simulink model "Grav_VarAeroBlock"  (R2016b)
settings: Solver=VariableStepAuto  StartTime=0.0  StopTime=10.0  RelTol=1e-3
undefined symbols (not defined in the file or in its folder): Sim
libraries: aerolibgravity2 x1
settings Model: Creator=rega0051  LastModifiedBy=rega0051
settings DataIOCC: SaveOutput=off  SignalLogging=off  DSMLogging=off  SaveTime=off

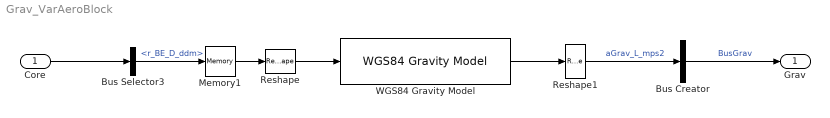
== system Grav_VarAeroBlock ==
  Core : Inport  OutDataTypeStr=Bus: BusCore
      settings: AttributesFormatString=%<OutDataTypeStr>
  Bus Creator : BusCreator  Inputs=1  OutDataTypeStr=Bus: BusGrav
      settings: AttributesFormatString=%<OutDataTypeStr>
  Bus Selector3 : BusSelector  OutputSignals=BusEom.r_BE_D_ddm
  Memory1 : Memory  X0=Sim.Trim.Init.rInit_BE_D_ddm  InheritSampleTime=on  LinearizeMemory=on  LinearizeAsDelay=on
      settings: AttributesFormatString=%<X0>
  Reshape : Reshape  OutputDimensions=3
  Reshape1 : Reshape  OutputDimensionality=Column vector (2-D)  OutputDimensions=[3,1]
  "WGS84 Gravity Model " : aerolibgravity2/WGS84 Gravity Model   model=WGS84 Taylor Series  units=Metric (MKS)  no_atmos=on  precessing=on  jd_loc=off  month=October  day=10  year=2004  no_centrifugal=on  action=Warning
  Grav : Outport  OutDataTypeStr=Bus: BusGrav
      settings: AttributesFormatString=%<OutDataTypeStr>
  wires:
  Memory1/1 -> Reshape/1
  Reshape/1 -> "WGS84 Gravity Model "/1
  Reshape1/1 -> Bus Creator/1  "aGrav_L_mps2"
  "WGS84 Gravity Model "/1 -> Reshape1/1
  Bus Selector3/1 -> Memory1/1  "<r_BE_D_ddm>"
  Core/1 -> Bus Selector3/1
  Bus Creator/1 -> Grav/1  "BusGrav"
